simulink model "backupSimulinkModels"  (R2020a)
settings: Solver=VariableStepAuto  StartTime=0.0  StopTime=10.0  RelTol=1e-3
libraries: aerolibutil x17, simulink x9, aerolibconvert2 x3
settings Model: Creator=rodrigo.weber  LastModifiedBy=rodrigo.weber

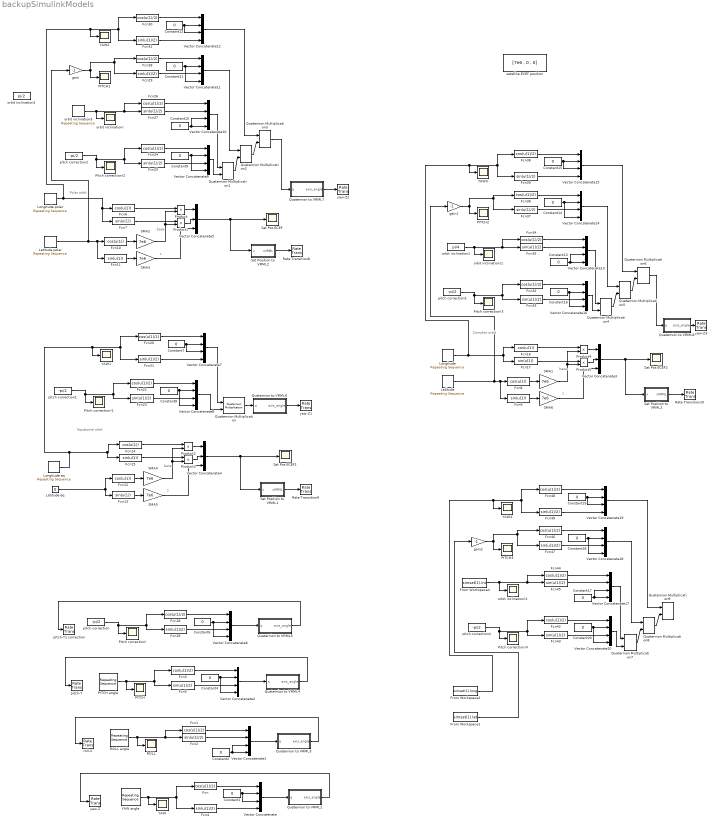
== system backupSimulinkModels ==
  note: z
  note: Equatorial orbit
  note: base
  note: z
  note: base
  note: Polar orbit
  note: base
  note: Complex orbit
  note: z
  Constant{1..2,4,6..20} (18 alike) : Constant  Value=0
  Fcn{,1,3,18,20,22,24,26,28,30,32,34,36,38,42,44,46,48} (18 alike) : Fcn  Expr=cos(u(1)/2)
  Fcn{6,8,10,12,14,16} (6 alike) : Fcn  Expr=cos(u(1))
  Fcn{7,9,11,13,15,17} (6 alike) : Fcn  Expr=sin(u(1))
  Fcn{2,4..5,19,21,23,25,27,29,31,33,35,37,39,43,45,47,49} (18 alike) : Fcn  Expr=sin(u(1)/2)
  From Workspace1 : FromWorkspace  VariableName=simsat(1).lat
  From Workspace2 : FromWorkspace  VariableName=simsat(1).long
  From Workspace4 : FromWorkspace  VariableName=simsat(1).inc
  Latitude : simulink/Sources/Repeating Sequence  rep_seq_t=[0 1e4 2e4 3e4 4e4]  rep_seq_y="[0   pi/4  0   -pi/4   0]"
  Latitude eq : Constant  Value=0
  Latitude polar : simulink/Sources/Repeating Sequence  rep_seq_t=[0 1e3 2e3 3e3 4e3]  rep_seq_y="[-pi/2   0   pi/2   0   -pi/2]"
  Longitude : simulink/Sources/Repeating Sequence  rep_seq_t=[0 1e4 2e4 3e4 4e4]  rep_seq_y="[0   pi/2   pi   1.5*pi   2*pi]"
  Longitude eq : simulink/Sources/Repeating Sequence  rep_seq_t=[0 1e4]  rep_seq_y=[0 2*pi]
  Longitude polar : simulink/Sources/Repeating Sequence  rep_seq_t="[0  2e3  2.001e3 4e3]"  rep_seq_y="[0   0   pi   pi ]"
  PITCH{,1..3} (4 alike) : Scope
  PITCH angle : simulink/Sources/Repeating Sequence  rep_seq_t=[0 1e4]  rep_seq_y=[-pi pi]
  Pitch correction!{,1..4} (5 alike) : Scope
  Product{,1..5} (6 alike) : Product
  Quaternion Multiplication{,1..9} (10 alike) : aerolibutil/Quaternion Multiplication
  Quaternion to VRML2 : Subsystem
  Quaternion to VRML3 : Subsystem
  Quaternion to VRML4 : Subsystem
  Quaternion to VRML5 : Subsystem
  Quaternion to VRML6 : Subsystem
  Quaternion to VRML7 : Subsystem
  Quaternion to VRML8 : Subsystem
  ROLL : Scope
  ROLL angle : simulink/Sources/Repeating Sequence  rep_seq_t=[0 1e4]  rep_seq_y=[-pi pi]
  Rate Transition10 : RateTransition
  Rate Transition8 : RateTransition
  Rate Transition9 : RateTransition
  SMA{1..6} (6 alike) : Gain  Gain=7e6
  Sat Pos ECEF : Scope
  Sat Pos ECEF1 : Scope
  Sat Pos ECEF2 : Scope
  Sat Position to VRML1 : Subsystem
  Sat Position to VRML2 : Subsystem
  Sat Position to VRML3 : Subsystem
  Vector Concatenate{,1..2,6..20} (18 alike) : Concatenate  NumInputs=4
  Vector Concatenate3 : Concatenate  NumInputs=3
  Vector Concatenate4 : Concatenate  NumInputs=3
  Vector Concatenate5 : Concatenate  NumInputs=3
  YAW{,1..4} (5 alike) : Scope
  YAW angle : simulink/Sources/Repeating Sequence  rep_seq_t=[0 1e4]  rep_seq_y=[-pi pi]
  gain : Gain  Gain=-1
  gain1 : Gain  Gain=-1
  gain2 : Gain  Gain=-1
  orbit inclination! : Scope
  orbit inclination!1 : Scope
  orbit inclination!2 : Scope
  orbit inclination1 : Constant  Value=pi/4
  orbit inclination2 : Constant  Value=pi/2
  orbit inclination3 : simulink/Sources/Repeating Sequence  rep_seq_t="[0  2e3  2.001e3 4e3]"  rep_seq_y="[pi/2   pi/2   -pi/2   -pi/2 ]"
  pitch correction{,1..4} (5 alike) : Constant  Value=-pi/2
  pitch-Y : RateTransition
  pitch-Y1 correction : RateTransition
  roll-X : RateTransition
  satellite ECEF position : Constant  Value=[7e6 , 0 , 0]  VectorParams1D=off
  yaw-Z{,1..3} (4 alike) : RateTransition
  wires:
  Product3/1 -> Vector Concatenate4/2
  Quaternion Multiplication/1 -> Quaternion to VRML6/1(q)
  Fcn22/1 -> Vector Concatenate8/1
  Fcn12/1 -> SMA4/1
  Fcn23/1 -> Vector Concatenate8/3
  Vector Concatenate8/1 -> Quaternion Multiplication/2
  Fcn13/1 -> SMA5/1
  SMA5/1 -> Vector Concatenate4/3
  Fcn20/1 -> Vector Concatenate7/1
  Vector Concatenate4/1 -> Sat Position to VRML1/1(x), Sat Pos ECEF1/1
  Quaternion to VRML6/1(axis_angle) -> yaw-Z1/1
  Constant7/1 -> Vector Concatenate7/2, Vector Concatenate7/3
  Longitude eq/1 -> Fcn15/1, Fcn14/1, YAW1/1, Fcn21/1, Fcn20/1
  Fcn21/1 -> Vector Concatenate7/4
  Constant8/1 -> Vector Concatenate8/4, Vector Concatenate8/2
  Fcn15/1 -> Product3/1
  SMA4/1 -> Product2/2, Product3/2
  Latitude eq/1 -> Fcn12/1, Fcn13/1
  Vector Concatenate7/1 -> Quaternion Multiplication/1
  Product2/1 -> Vector Concatenate4/1
  pitch correction1/1 -> Pitch correction!1/1, Fcn23/1, Fcn22/1
  Fcn14/1 -> Product2/1
  Sat Position to VRML1/1(xVRML) -> Rate Transition9/1
  Fcn6/1 -> Product/1
  Product1/1 -> Vector Concatenate5/2
  Vector Concatenate5/1 -> Sat Position to VRML2/1(x), Sat Pos ECEF/1
  Vector Concatenate9/1 -> Quaternion Multiplication1/2
  Fcn10/1 -> SMA2/1
  Quaternion Multiplication3/1 -> Quaternion to VRML7/1(q)
  Longitude polar/1 -> YAW2/1, Fcn31/1, Fcn30/1, Fcn7/1, Fcn6/1
  Constant12/1 -> Vector Concatenate12/2, Vector Concatenate12/3
  Fcn31/1 -> Vector Concatenate12/4
  Vector Concatenate11/1 -> Quaternion Multiplication2/1
  orbit inclination3/1 -> orbit inclination!/1, Fcn27/1, Fcn26/1
  Fcn29/1 -> Vector Concatenate11/3
  Constant11/1 -> Vector Concatenate11/4, Vector Concatenate11/2
  Quaternion Multiplication1/1 -> Quaternion Multiplication2/2
  Fcn27/1 -> Vector Concatenate10/2
  Vector Concatenate10/1 -> Quaternion Multiplication1/1
  Fcn30/1 -> Vector Concatenate12/1
  Latitude polar/1 -> gain/1, Fcn11/1, Fcn10/1
  Sat Position to VRML2/1(xVRML) -> Rate Transition8/1
  Fcn24/1 -> Vector Concatenate9/1
  Quaternion to VRML7/1(axis_angle) -> yaw-Z2/1
  Constant9/1 -> Vector Concatenate9/4, Vector Concatenate9/2
  Constant10/1 -> Vector Concatenate10/3, Vector Concatenate10/4
  Quaternion Multiplication2/1 -> Quaternion Multiplication3/2
  Fcn26/1 -> Vector Concatenate10/1
  pitch correction2/1 -> Pitch correction!2/1, Fcn25/1, Fcn24/1
  Vector Concatenate12/1 -> Quaternion Multiplication3/1
  Fcn25/1 -> Vector Concatenate9/3
  Fcn28/1 -> Vector Concatenate11/1
  SMA3/1 -> Vector Concatenate5/3
  gain/1 -> Fcn28/1, Fcn29/1, PITCH1/1
  Fcn7/1 -> Product1/1
  Product/1 -> Vector Concatenate5/1
  Fcn11/1 -> SMA3/1
  SMA2/1 -> Product/2, Product1/2
  SMA1/1 -> Product4/2, Product5/2
  orbit inclination1/1 -> orbit inclination!1/1, Fcn35/1, Fcn34/1
  Quaternion Multiplication6/1 -> Quaternion to VRML8/1(q)
  Vector Concatenate13/1 -> Quaternion Multiplication4/1
  Fcn38/1 -> Vector Concatenate15/1
  Constant13/1 -> Vector Concatenate13/3, Vector Concatenate13/4
  Quaternion Multiplication5/1 -> Quaternion Multiplication6/2
  Quaternion Multiplication4/1 -> Quaternion Multiplication5/2
  Longitude/1 -> YAW3/1, Fcn39/1, Fcn38/1, Fcn17/1, Fcn16/1
  Quaternion to VRML8/1(axis_angle) -> yaw-Z3/1
  Constant14/1 -> Vector Concatenate14/4, Vector Concatenate14/2
  Fcn37/1 -> Vector Concatenate14/3
  pitch correction3/1 -> Pitch correction!3/1, Fcn33/1, Fcn32/1
  Vector Concatenate16/1 -> Quaternion Multiplication4/2
  Fcn9/1 -> SMA6/1
  Fcn36/1 -> Vector Concatenate14/1
  Vector Concatenate15/1 -> Quaternion Multiplication6/1
  Fcn33/1 -> Vector Concatenate16/3
  Fcn32/1 -> Vector Concatenate16/1
  Fcn35/1 -> Vector Concatenate13/2
  Vector Concatenate14/1 -> Quaternion Multiplication5/1
  Fcn34/1 -> Vector Concatenate13/1
  Fcn39/1 -> Vector Concatenate15/4
  Product5/1 -> Vector Concatenate3/2
  Fcn16/1 -> Product4/1
  Sat Position to VRML3/1(xVRML) -> Rate Transition10/1
  gain1/1 -> Fcn36/1, Fcn37/1, PITCH2/1
  Fcn17/1 -> Product5/1
  SMA6/1 -> Vector Concatenate3/3
  Constant15/1 -> Vector Concatenate15/2, Vector Concatenate15/3
  Constant16/1 -> Vector Concatenate16/4, Vector Concatenate16/2
  Vector Concatenate3/1 -> Sat Position to VRML3/1(x), Sat Pos ECEF2/1
  Product4/1 -> Vector Concatenate3/1
  Latitude/1 -> gain1/1, Fcn9/1, Fcn8/1
  Fcn8/1 -> SMA1/1
  Fcn48/1 -> Vector Concatenate19/1
  Fcn46/1 -> Vector Concatenate18/1
  Vector Concatenate20/1 -> Quaternion Multiplication7/2
  Fcn44/1 -> Vector Concatenate17/1
  Vector Concatenate19/1 -> Quaternion Multiplication9/1
  Quaternion Multiplication8/1 -> Quaternion Multiplication9/2
  Fcn49/1 -> Vector Concatenate19/4
  Fcn43/1 -> Vector Concatenate20/3
  Vector Concatenate18/1 -> Quaternion Multiplication8/1
  From Workspace1/1 -> gain2/1
  Fcn45/1 -> Vector Concatenate17/2
  Fcn47/1 -> Vector Concatenate18/3
  Constant18/1 -> Vector Concatenate18/4, Vector Concatenate18/2
  Quaternion Multiplication7/1 -> Quaternion Multiplication8/2
  Constant20/1 -> Vector Concatenate20/4, Vector Concatenate20/2
  Constant19/1 -> Vector Concatenate19/2, Vector Concatenate19/3
  From Workspace4/1 -> orbit inclination!2/1, Fcn45/1, Fcn44/1
  Vector Concatenate17/1 -> Quaternion Multiplication7/1
  Constant17/1 -> Vector Concatenate17/3, Vector Concatenate17/4
  pitch correction4/1 -> Pitch correction!4/1, Fcn43/1, Fcn42/1
  gain2/1 -> Fcn46/1, Fcn47/1, PITCH3/1
  From Workspace2/1 -> YAW4/1, Fcn49/1, Fcn48/1
  Fcn42/1 -> Vector Concatenate20/1
  Vector Concatenate6/1 -> Quaternion to VRML5/1(q)
  Fcn3/1 -> Vector Concatenate2/1
  Constant2/1 -> Vector Concatenate1/3, Vector Concatenate1/4
  ROLL angle/1 -> ROLL/1, Fcn2/1, Fcn1/1
  Constant1/1 -> Vector Concatenate/2, Vector Concatenate/3
  Quaternion to VRML5/1(axis_angle) -> pitch-Y1 correction/1
  Fcn18/1 -> Vector Concatenate6/1
  Fcn1/1 -> Vector Concatenate1/1
  Fcn19/1 -> Vector Concatenate6/3
  Fcn/1 -> Vector Concatenate/1
  Fcn5/1 -> Vector Concatenate2/3
  Quaternion to VRML2/1(axis_angle) -> yaw-Z/1
  Constant6/1 -> Vector Concatenate6/4, Vector Concatenate6/2
  YAW angle/1 -> YAW/1, Fcn4/1, Fcn/1
  Vector Concatenate1/1 -> Quaternion to VRML3/1(q)
  Fcn4/1 -> Vector Concatenate/4
  Fcn2/1 -> Vector Concatenate1/2
  Quaternion to VRML3/1(axis_angle) -> roll-X/1
  Vector Concatenate2/1 -> Quaternion to VRML4/1(q)
  PITCH angle/1 -> PITCH/1, Fcn5/1, Fcn3/1
  Quaternion to VRML4/1(axis_angle) -> pitch-Y/1
  pitch correction/1 -> Pitch correction!/1, Fcn19/1, Fcn18/1
  Constant4/1 -> Vector Concatenate2/4, Vector Concatenate2/2
  Vector Concatenate/1 -> Quaternion to VRML2/1(q)

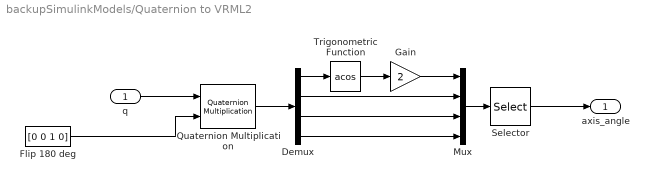
== system backupSimulinkModels/Quaternion to VRML2 ==
  q : Inport
  Demux : Demux
  Flip 180 deg : Constant  Value=[0 0 1 0]
  Gain : Gain  Gain=2
  Mux : Mux
  Quaternion Multiplication : aerolibutil/Quaternion Multiplication
  Selector : Selector  InputPortWidth=4  IndexOptions=Index vector (dialog)  Indices=[3 4 2 1]  OutputSizes=1
  Trigonometric Function : Trigonometry  Operator=acos
  axis_angle : Outport  VectorParamsAs1DForOutWhenUnconnected=off
  wires:
  Demux/4 -> Mux/4
  Demux/3 -> Mux/3
  Demux/2 -> Mux/2
  Gain/1 -> Mux/1
  Selector/1 -> axis_angle/1
  q/1 -> Quaternion Multiplication/1
  Mux/1 -> Selector/1
  Trigonometric Function/1 -> Gain/1
  Demux/1 -> Trigonometric Function/1
  Flip 180 deg/1 -> Quaternion Multiplication/2
  Quaternion Multiplication/1 -> Demux/1

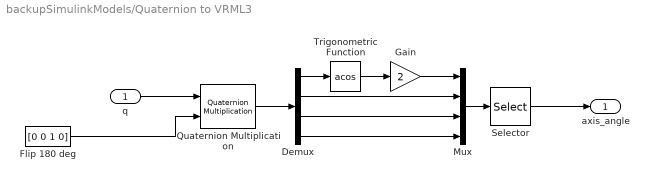
== system backupSimulinkModels/Quaternion to VRML3 ==
  q : Inport
  Demux : Demux
  Flip 180 deg : Constant  Value=[0 0 1 0]
  Gain : Gain  Gain=2
  Mux : Mux
  Quaternion Multiplication : aerolibutil/Quaternion Multiplication
  Selector : Selector  InputPortWidth=4  IndexOptions=Index vector (dialog)  Indices=[3 4 2 1]  OutputSizes=1
  Trigonometric Function : Trigonometry  Operator=acos
  axis_angle : Outport  VectorParamsAs1DForOutWhenUnconnected=off
  wires:
  Demux/4 -> Mux/4
  Demux/3 -> Mux/3
  Demux/2 -> Mux/2
  Gain/1 -> Mux/1
  Selector/1 -> axis_angle/1
  q/1 -> Quaternion Multiplication/1
  Mux/1 -> Selector/1
  Trigonometric Function/1 -> Gain/1
  Demux/1 -> Trigonometric Function/1
  Flip 180 deg/1 -> Quaternion Multiplication/2
  Quaternion Multiplication/1 -> Demux/1

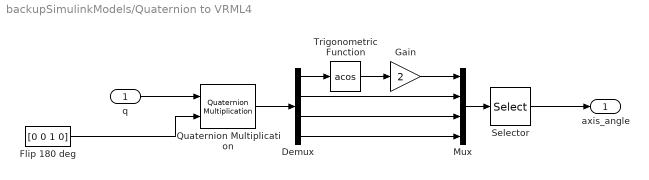
== system backupSimulinkModels/Quaternion to VRML4 ==
  q : Inport
  Demux : Demux
  Flip 180 deg : Constant  Value=[0 0 1 0]
  Gain : Gain  Gain=2
  Mux : Mux
  Quaternion Multiplication : aerolibutil/Quaternion Multiplication
  Selector : Selector  InputPortWidth=4  IndexOptions=Index vector (dialog)  Indices=[3 4 2 1]  OutputSizes=1
  Trigonometric Function : Trigonometry  Operator=acos
  axis_angle : Outport  VectorParamsAs1DForOutWhenUnconnected=off
  wires:
  Demux/4 -> Mux/4
  Demux/3 -> Mux/3
  Demux/2 -> Mux/2
  Gain/1 -> Mux/1
  Selector/1 -> axis_angle/1
  q/1 -> Quaternion Multiplication/1
  Mux/1 -> Selector/1
  Trigonometric Function/1 -> Gain/1
  Demux/1 -> Trigonometric Function/1
  Flip 180 deg/1 -> Quaternion Multiplication/2
  Quaternion Multiplication/1 -> Demux/1

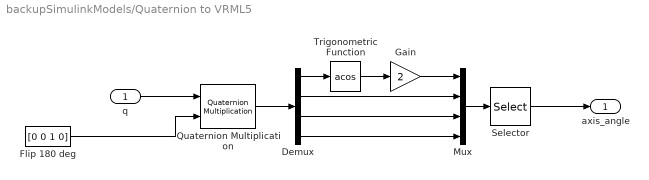
== system backupSimulinkModels/Quaternion to VRML5 ==
  q : Inport
  Demux : Demux
  Flip 180 deg : Constant  Value=[0 0 1 0]
  Gain : Gain  Gain=2
  Mux : Mux
  Quaternion Multiplication : aerolibutil/Quaternion Multiplication
  Selector : Selector  InputPortWidth=4  IndexOptions=Index vector (dialog)  Indices=[3 4 2 1]  OutputSizes=1
  Trigonometric Function : Trigonometry  Operator=acos
  axis_angle : Outport  VectorParamsAs1DForOutWhenUnconnected=off
  wires:
  Demux/4 -> Mux/4
  Demux/3 -> Mux/3
  Demux/2 -> Mux/2
  Gain/1 -> Mux/1
  Selector/1 -> axis_angle/1
  q/1 -> Quaternion Multiplication/1
  Mux/1 -> Selector/1
  Trigonometric Function/1 -> Gain/1
  Demux/1 -> Trigonometric Function/1
  Flip 180 deg/1 -> Quaternion Multiplication/2
  Quaternion Multiplication/1 -> Demux/1

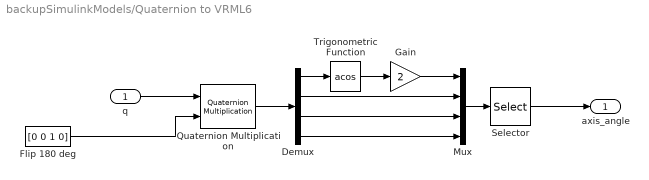
== system backupSimulinkModels/Quaternion to VRML6 ==
  q : Inport
  Demux : Demux
  Flip 180 deg : Constant  Value=[0 0 1 0]
  Gain : Gain  Gain=2
  Mux : Mux
  Quaternion Multiplication : aerolibutil/Quaternion Multiplication
  Selector : Selector  InputPortWidth=4  IndexOptions=Index vector (dialog)  Indices=[3 4 2 1]  OutputSizes=1
  Trigonometric Function : Trigonometry  Operator=acos
  axis_angle : Outport  VectorParamsAs1DForOutWhenUnconnected=off
  wires:
  Demux/4 -> Mux/4
  Demux/3 -> Mux/3
  Demux/2 -> Mux/2
  Gain/1 -> Mux/1
  Selector/1 -> axis_angle/1
  q/1 -> Quaternion Multiplication/1
  Mux/1 -> Selector/1
  Trigonometric Function/1 -> Gain/1
  Demux/1 -> Trigonometric Function/1
  Flip 180 deg/1 -> Quaternion Multiplication/2
  Quaternion Multiplication/1 -> Demux/1

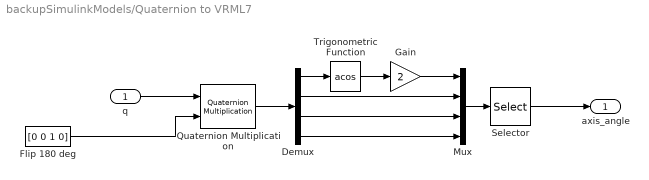
== system backupSimulinkModels/Quaternion to VRML7 ==
  q : Inport
  Demux : Demux
  Flip 180 deg : Constant  Value=[0 0 1 0]
  Gain : Gain  Gain=2
  Mux : Mux
  Quaternion Multiplication : aerolibutil/Quaternion Multiplication
  Selector : Selector  InputPortWidth=4  IndexOptions=Index vector (dialog)  Indices=[3 4 2 1]  OutputSizes=1
  Trigonometric Function : Trigonometry  Operator=acos
  axis_angle : Outport  VectorParamsAs1DForOutWhenUnconnected=off
  wires:
  Demux/4 -> Mux/4
  Demux/3 -> Mux/3
  Demux/2 -> Mux/2
  Gain/1 -> Mux/1
  Selector/1 -> axis_angle/1
  Mux/1 -> Selector/1
  Trigonometric Function/1 -> Gain/1
  Demux/1 -> Trigonometric Function/1
  Flip 180 deg/1 -> Quaternion Multiplication/2
  q/1 -> Quaternion Multiplication/1
  Quaternion Multiplication/1 -> Demux/1

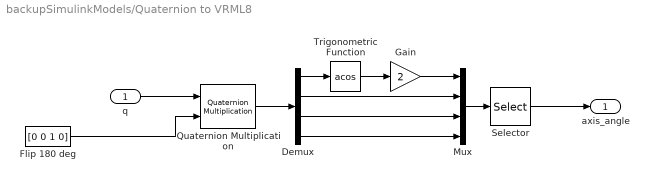
== system backupSimulinkModels/Quaternion to VRML8 ==
  q : Inport
  Demux : Demux
  Flip 180 deg : Constant  Value=[0 0 1 0]
  Gain : Gain  Gain=2
  Mux : Mux
  Quaternion Multiplication : aerolibutil/Quaternion Multiplication
  Selector : Selector  InputPortWidth=4  IndexOptions=Index vector (dialog)  Indices=[3 4 2 1]  OutputSizes=1
  Trigonometric Function : Trigonometry  Operator=acos
  axis_angle : Outport  VectorParamsAs1DForOutWhenUnconnected=off
  wires:
  Demux/4 -> Mux/4
  Demux/3 -> Mux/3
  Demux/2 -> Mux/2
  Gain/1 -> Mux/1
  Selector/1 -> axis_angle/1
  Mux/1 -> Selector/1
  Trigonometric Function/1 -> Gain/1
  Demux/1 -> Trigonometric Function/1
  Flip 180 deg/1 -> Quaternion Multiplication/2
  q/1 -> Quaternion Multiplication/1
  Quaternion Multiplication/1 -> Demux/1

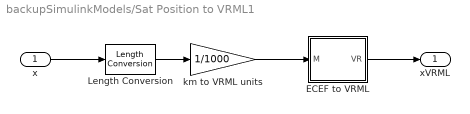
== system backupSimulinkModels/Sat Position to VRML1 ==
  x : Inport
  ECEF to VRML : Subsystem
  Length Conversion : aerolibconvert2/Length Conversion  IU=m  OU=km
  km to VRML units : Gain  Gain=1/1000
  xVRML : Outport  VectorParamsAs1DForOutWhenUnconnected=off
  wires:
  ECEF to VRML/1(VR) -> xVRML/1
  x/1 -> Length Conversion/1
  km to VRML units/1 -> ECEF to VRML/1(M)
  Length Conversion/1 -> km to VRML units/1

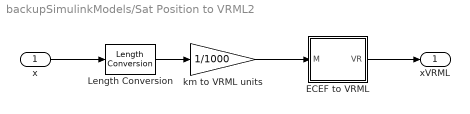
== system backupSimulinkModels/Sat Position to VRML2 ==
  x : Inport
  ECEF to VRML : Subsystem
  Length Conversion : aerolibconvert2/Length Conversion  IU=m  OU=km
  km to VRML units : Gain  Gain=1/1000
  xVRML : Outport  VectorParamsAs1DForOutWhenUnconnected=off
  wires:
  ECEF to VRML/1(VR) -> xVRML/1
  x/1 -> Length Conversion/1
  km to VRML units/1 -> ECEF to VRML/1(M)
  Length Conversion/1 -> km to VRML units/1

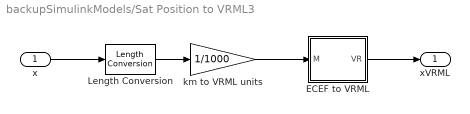
== system backupSimulinkModels/Sat Position to VRML3 ==
  x : Inport
  ECEF to VRML : Subsystem
  Length Conversion : aerolibconvert2/Length Conversion  IU=m  OU=km
  km to VRML units : Gain  Gain=1/1000
  xVRML : Outport  VectorParamsAs1DForOutWhenUnconnected=off
  wires:
  ECEF to VRML/1(VR) -> xVRML/1
  x/1 -> Length Conversion/1
  km to VRML units/1 -> ECEF to VRML/1(M)
  Length Conversion/1 -> km to VRML units/1

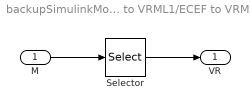
== system backupSimulinkModels/Sat Position to VRML1/ECEF to VRML ==
  M : Inport  PortDimensions=3
  Selector : Selector  InputPortWidth=3  IndexOptions=Index vector (dialog)  Indices=[2 3 1]  OutputSizes=1
  VR : Outport  PortDimensions=3  VectorParamsAs1DForOutWhenUnconnected=off
  wires:
  M/1 -> Selector/1
  Selector/1 -> VR/1

== system backupSimulinkModels/Sat Position to VRML2/ECEF to VRML ==
  M : Inport  PortDimensions=3
  Selector : Selector  InputPortWidth=3  IndexOptions=Index vector (dialog)  Indices=[2 3 1]  OutputSizes=1
  VR : Outport  PortDimensions=3  VectorParamsAs1DForOutWhenUnconnected=off
  wires:
  M/1 -> Selector/1
  Selector/1 -> VR/1

== system backupSimulinkModels/Sat Position to VRML3/ECEF to VRML ==
  M : Inport  PortDimensions=3
  Selector : Selector  InputPortWidth=3  IndexOptions=Index vector (dialog)  Indices=[2 3 1]  OutputSizes=1
  VR : Outport  PortDimensions=3  VectorParamsAs1DForOutWhenUnconnected=off
  wires:
  M/1 -> Selector/1
  Selector/1 -> VR/1
